simulink model "LV_grid"  (R2021b)
settings: Solver=VariableStepAuto  StartTime=0  StopTime=5.0005  FixedStep=5e-4  RelTol=1e-3
model workspace (MAT data in the model file):
  P2_1 = 3450
  idx = 1
  time_counter = 1
libraries: spsGroundLib x97, spsStairGeneratorLib x96, spsPiSectionLineLib x90, spsThreePhasePISectionLineLib x90, spsVariableInductorLib x48, spsVariableResistorLib x48, spsRMSLib x36, spsThreePhaseVIMeasurementLib x34, spsACVoltageSourceLib x5, spsLinearTransformerLib x5, spsPower3phInstantaneousLib x1, spsThreePhaseMutualInductanceZ1Z0Lib x1
(part 4 of 6)

== system LV_grid/L10/L2 ==
  Pi Section Line : spsPiSectionLineLib/Pi Section Line  LConnTagsString=__new0  RConnTagsString=__new0  Phases=1  PiSections=1  Length=0.0025  Frequency=50  Resistance=0.274  Inductance=0.073  Capacitance=12.74e-9  Measurements=None  Measurements2=None
      settings: SourceProductBaseCode=PS
  Three-Phase PI Section Line : spsThreePhasePISectionLineLib/Three-Phase PI Section Line  LConnTagsString=a|b|c  RConnTagsString=A|B|C  Length=0.0025  Frequency=50  Resistances=[ 0.274 0.959]  Inductances=[ 0.073 0.079]  Capacitances=[12.74e-9 7.751e-9]
  A : PMIOPort  Side=Left
  B : PMIOPort  Port=2  Side=Left
  C : PMIOPort  Port=3  Side=Left
  N : PMIOPort  Port=4  Side=Left
  a : PMIOPort  Port=5  Side=Right
  b : PMIOPort  Port=6  Side=Right
  c : PMIOPort  Port=7  Side=Right
  n : PMIOPort  Port=8  Side=Right
  connections:
  Pi Section Line/LConn1 -- N/RConn1
  Pi Section Line/RConn1 -- n/RConn1
  C/RConn1 -- Three-Phase PI Section Line/LConn3
  B/RConn1 -- Three-Phase PI Section Line/LConn2
  A/RConn1 -- Three-Phase PI Section Line/LConn1
  Three-Phase PI Section Line/RConn3 -- c/RConn1
  Three-Phase PI Section Line/RConn2 -- b/RConn1
  Three-Phase PI Section Line/RConn1 -- a/RConn1

== system LV_grid/L11/L1 ==
  Pi Section Line : spsPiSectionLineLib/Pi Section Line  LConnTagsString=__new0  RConnTagsString=__new0  Phases=1  PiSections=1  Length=0.0025  Frequency=50  Resistance=0.274  Inductance=0.073  Capacitance=12.74e-9  Measurements=None  Measurements2=None
      settings: SourceProductBaseCode=PS
  Three-Phase PI Section Line : spsThreePhasePISectionLineLib/Three-Phase PI Section Line  LConnTagsString=a|b|c  RConnTagsString=A|B|C  Length=0.0025  Frequency=50  Resistances=[ 0.274 0.959]  Inductances=[ 0.073 0.079]  Capacitances=[12.74e-9 7.751e-9]
  A : PMIOPort  Side=Left
  B : PMIOPort  Port=2  Side=Left
  C : PMIOPort  Port=3  Side=Left
  N : PMIOPort  Port=4  Side=Left
  a : PMIOPort  Port=5  Side=Right
  b : PMIOPort  Port=6  Side=Right
  c : PMIOPort  Port=7  Side=Right
  n : PMIOPort  Port=8  Side=Right
  connections:
  Pi Section Line/LConn1 -- N/RConn1
  Pi Section Line/RConn1 -- n/RConn1
  C/RConn1 -- Three-Phase PI Section Line/LConn3
  B/RConn1 -- Three-Phase PI Section Line/LConn2
  A/RConn1 -- Three-Phase PI Section Line/LConn1
  Three-Phase PI Section Line/RConn3 -- c/RConn1
  Three-Phase PI Section Line/RConn2 -- b/RConn1
  Three-Phase PI Section Line/RConn1 -- a/RConn1

== system LV_grid/L11/L2 ==
  Pi Section Line : spsPiSectionLineLib/Pi Section Line  LConnTagsString=__new0  RConnTagsString=__new0  Phases=1  PiSections=1  Length=0.0025  Frequency=50  Resistance=0.274  Inductance=0.073  Capacitance=12.74e-9  Measurements=None  Measurements2=None
      settings: SourceProductBaseCode=PS
  Three-Phase PI Section Line : spsThreePhasePISectionLineLib/Three-Phase PI Section Line  LConnTagsString=a|b|c  RConnTagsString=A|B|C  Length=0.0025  Frequency=50  Resistances=[ 0.274 0.959]  Inductances=[ 0.073 0.079]  Capacitances=[12.74e-9 7.751e-9]
  A : PMIOPort  Side=Left
  B : PMIOPort  Port=2  Side=Left
  C : PMIOPort  Port=3  Side=Left
  N : PMIOPort  Port=4  Side=Left
  a : PMIOPort  Port=5  Side=Right
  b : PMIOPort  Port=6  Side=Right
  c : PMIOPort  Port=7  Side=Right
  n : PMIOPort  Port=8  Side=Right
  connections:
  Pi Section Line/LConn1 -- N/RConn1
  Pi Section Line/RConn1 -- n/RConn1
  C/RConn1 -- Three-Phase PI Section Line/LConn3
  B/RConn1 -- Three-Phase PI Section Line/LConn2
  A/RConn1 -- Three-Phase PI Section Line/LConn1
  Three-Phase PI Section Line/RConn3 -- c/RConn1
  Three-Phase PI Section Line/RConn2 -- b/RConn1
  Three-Phase PI Section Line/RConn1 -- a/RConn1

== system LV_grid/L12/L1 ==
  Pi Section Line : spsPiSectionLineLib/Pi Section Line  LConnTagsString=__new0  RConnTagsString=__new0  Phases=1  PiSections=1  Length=0.0025  Frequency=50  Resistance=0.274  Inductance=0.073  Capacitance=12.74e-9  Measurements=None  Measurements2=None
      settings: SourceProductBaseCode=PS
  Three-Phase PI Section Line : spsThreePhasePISectionLineLib/Three-Phase PI Section Line  LConnTagsString=a|b|c  RConnTagsString=A|B|C  Length=0.0025  Frequency=50  Resistances=[ 0.274 0.959]  Inductances=[ 0.073 0.079]  Capacitances=[12.74e-9 7.751e-9]
  A : PMIOPort  Side=Left
  B : PMIOPort  Port=2  Side=Left
  C : PMIOPort  Port=3  Side=Left
  N : PMIOPort  Port=4  Side=Left
  a : PMIOPort  Port=5  Side=Right
  b : PMIOPort  Port=6  Side=Right
  c : PMIOPort  Port=7  Side=Right
  n : PMIOPort  Port=8  Side=Right
  connections:
  Pi Section Line/LConn1 -- N/RConn1
  Pi Section Line/RConn1 -- n/RConn1
  C/RConn1 -- Three-Phase PI Section Line/LConn3
  B/RConn1 -- Three-Phase PI Section Line/LConn2
  A/RConn1 -- Three-Phase PI Section Line/LConn1
  Three-Phase PI Section Line/RConn3 -- c/RConn1
  Three-Phase PI Section Line/RConn2 -- b/RConn1
  Three-Phase PI Section Line/RConn1 -- a/RConn1

== system LV_grid/L12/L2 ==
  Pi Section Line : spsPiSectionLineLib/Pi Section Line  LConnTagsString=__new0  RConnTagsString=__new0  Phases=1  PiSections=1  Length=0.0025  Frequency=50  Resistance=0.274  Inductance=0.073  Capacitance=12.74e-9  Measurements=None  Measurements2=None
      settings: SourceProductBaseCode=PS
  Three-Phase PI Section Line : spsThreePhasePISectionLineLib/Three-Phase PI Section Line  LConnTagsString=a|b|c  RConnTagsString=A|B|C  Length=0.0025  Frequency=50  Resistances=[ 0.274 0.959]  Inductances=[ 0.073 0.079]  Capacitances=[12.74e-9 7.751e-9]
  A : PMIOPort  Side=Left
  B : PMIOPort  Port=2  Side=Left
  C : PMIOPort  Port=3  Side=Left
  N : PMIOPort  Port=4  Side=Left
  a : PMIOPort  Port=5  Side=Right
  b : PMIOPort  Port=6  Side=Right
  c : PMIOPort  Port=7  Side=Right
  n : PMIOPort  Port=8  Side=Right
  connections:
  Pi Section Line/LConn1 -- N/RConn1
  Pi Section Line/RConn1 -- n/RConn1
  C/RConn1 -- Three-Phase PI Section Line/LConn3
  B/RConn1 -- Three-Phase PI Section Line/LConn2
  A/RConn1 -- Three-Phase PI Section Line/LConn1
  Three-Phase PI Section Line/RConn3 -- c/RConn1
  Three-Phase PI Section Line/RConn2 -- b/RConn1
  Three-Phase PI Section Line/RConn1 -- a/RConn1

== system LV_grid/L12/L3 ==
  Pi Section Line : spsPiSectionLineLib/Pi Section Line  LConnTagsString=__new0  RConnTagsString=__new0  Phases=1  PiSections=1  Length=0.0025  Frequency=50  Resistance=0.274  Inductance=0.073  Capacitance=12.74e-9  Measurements=None  Measurements2=None
      settings: SourceProductBaseCode=PS
  Three-Phase PI Section Line : spsThreePhasePISectionLineLib/Three-Phase PI Section Line  LConnTagsString=a|b|c  RConnTagsString=A|B|C  Length=0.0025  Frequency=50  Resistances=[ 0.274 0.959]  Inductances=[ 0.073 0.079]  Capacitances=[12.74e-9 7.751e-9]
  A : PMIOPort  Side=Left
  B : PMIOPort  Port=2  Side=Left
  C : PMIOPort  Port=3  Side=Left
  N : PMIOPort  Port=4  Side=Left
  a : PMIOPort  Port=5  Side=Right
  b : PMIOPort  Port=6  Side=Right
  c : PMIOPort  Port=7  Side=Right
  n : PMIOPort  Port=8  Side=Right
  connections:
  Pi Section Line/LConn1 -- N/RConn1
  Pi Section Line/RConn1 -- n/RConn1
  C/RConn1 -- Three-Phase PI Section Line/LConn3
  B/RConn1 -- Three-Phase PI Section Line/LConn2
  A/RConn1 -- Three-Phase PI Section Line/LConn1
  Three-Phase PI Section Line/RConn3 -- c/RConn1
  Three-Phase PI Section Line/RConn2 -- b/RConn1
  Three-Phase PI Section Line/RConn1 -- a/RConn1

== system LV_grid/L12/L4 ==
  Pi Section Line : spsPiSectionLineLib/Pi Section Line  LConnTagsString=__new0  RConnTagsString=__new0  Phases=1  PiSections=1  Length=0.0025  Frequency=50  Resistance=0.274  Inductance=0.073  Capacitance=12.74e-9  Measurements=None  Measurements2=None
      settings: SourceProductBaseCode=PS
  Three-Phase PI Section Line : spsThreePhasePISectionLineLib/Three-Phase PI Section Line  LConnTagsString=a|b|c  RConnTagsString=A|B|C  Length=0.0025  Frequency=50  Resistances=[ 0.274 0.959]  Inductances=[ 0.073 0.079]  Capacitances=[12.74e-9 7.751e-9]
  A : PMIOPort  Side=Left
  B : PMIOPort  Port=2  Side=Left
  C : PMIOPort  Port=3  Side=Left
  N : PMIOPort  Port=4  Side=Left
  a : PMIOPort  Port=5  Side=Right
  b : PMIOPort  Port=6  Side=Right
  c : PMIOPort  Port=7  Side=Right
  n : PMIOPort  Port=8  Side=Right
  connections:
  Pi Section Line/LConn1 -- N/RConn1
  Pi Section Line/RConn1 -- n/RConn1
  C/RConn1 -- Three-Phase PI Section Line/LConn3
  B/RConn1 -- Three-Phase PI Section Line/LConn2
  A/RConn1 -- Three-Phase PI Section Line/LConn1
  Three-Phase PI Section Line/RConn3 -- c/RConn1
  Three-Phase PI Section Line/RConn2 -- b/RConn1
  Three-Phase PI Section Line/RConn1 -- a/RConn1

== system LV_grid/L12/L5 ==
  Pi Section Line : spsPiSectionLineLib/Pi Section Line  LConnTagsString=__new0  RConnTagsString=__new0  Phases=1  PiSections=1  Length=0.0025  Frequency=50  Resistance=0.274  Inductance=0.073  Capacitance=12.74e-9  Measurements=None  Measurements2=None
      settings: SourceProductBaseCode=PS
  Three-Phase PI Section Line : spsThreePhasePISectionLineLib/Three-Phase PI Section Line  LConnTagsString=a|b|c  RConnTagsString=A|B|C  Length=0.0025  Frequency=50  Resistances=[ 0.274 0.959]  Inductances=[ 0.073 0.079]  Capacitances=[12.74e-9 7.751e-9]
  A : PMIOPort  Side=Left
  B : PMIOPort  Port=2  Side=Left
  C : PMIOPort  Port=3  Side=Left
  N : PMIOPort  Port=4  Side=Left
  a : PMIOPort  Port=5  Side=Right
  b : PMIOPort  Port=6  Side=Right
  c : PMIOPort  Port=7  Side=Right
  n : PMIOPort  Port=8  Side=Right
  connections:
  Pi Section Line/LConn1 -- N/RConn1
  Pi Section Line/RConn1 -- n/RConn1
  C/RConn1 -- Three-Phase PI Section Line/LConn3
  B/RConn1 -- Three-Phase PI Section Line/LConn2
  A/RConn1 -- Three-Phase PI Section Line/LConn1
  Three-Phase PI Section Line/RConn3 -- c/RConn1
  Three-Phase PI Section Line/RConn2 -- b/RConn1
  Three-Phase PI Section Line/RConn1 -- a/RConn1

== system LV_grid/L13/L1 ==
  Pi Section Line : spsPiSectionLineLib/Pi Section Line  LConnTagsString=__new0  RConnTagsString=__new0  Phases=1  PiSections=1  Length=0.0025  Frequency=50  Resistance=0.274  Inductance=0.073  Capacitance=12.74e-9  Measurements=None  Measurements2=None
      settings: SourceProductBaseCode=PS
  Three-Phase PI Section Line : spsThreePhasePISectionLineLib/Three-Phase PI Section Line  LConnTagsString=a|b|c  RConnTagsString=A|B|C  Length=0.0025  Frequency=50  Resistances=[ 0.274 0.959]  Inductances=[ 0.073 0.079]  Capacitances=[12.74e-9 7.751e-9]
  A : PMIOPort  Side=Left
  B : PMIOPort  Port=2  Side=Left
  C : PMIOPort  Port=3  Side=Left
  N : PMIOPort  Port=4  Side=Left
  a : PMIOPort  Port=5  Side=Right
  b : PMIOPort  Port=6  Side=Right
  c : PMIOPort  Port=7  Side=Right
  n : PMIOPort  Port=8  Side=Right
  connections:
  Pi Section Line/LConn1 -- N/RConn1
  Pi Section Line/RConn1 -- n/RConn1
  C/RConn1 -- Three-Phase PI Section Line/LConn3
  B/RConn1 -- Three-Phase PI Section Line/LConn2
  A/RConn1 -- Three-Phase PI Section Line/LConn1
  Three-Phase PI Section Line/RConn3 -- c/RConn1
  Three-Phase PI Section Line/RConn2 -- b/RConn1
  Three-Phase PI Section Line/RConn1 -- a/RConn1

== system LV_grid/L13/L2 ==
  Pi Section Line : spsPiSectionLineLib/Pi Section Line  LConnTagsString=__new0  RConnTagsString=__new0  Phases=1  PiSections=1  Length=0.0025  Frequency=50  Resistance=0.274  Inductance=0.073  Capacitance=12.74e-9  Measurements=None  Measurements2=None
      settings: SourceProductBaseCode=PS
  Three-Phase PI Section Line : spsThreePhasePISectionLineLib/Three-Phase PI Section Line  LConnTagsString=a|b|c  RConnTagsString=A|B|C  Length=0.0025  Frequency=50  Resistances=[ 0.274 0.959]  Inductances=[ 0.073 0.079]  Capacitances=[12.74e-9 7.751e-9]
  A : PMIOPort  Side=Left
  B : PMIOPort  Port=2  Side=Left
  C : PMIOPort  Port=3  Side=Left
  N : PMIOPort  Port=4  Side=Left
  a : PMIOPort  Port=5  Side=Right
  b : PMIOPort  Port=6  Side=Right
  c : PMIOPort  Port=7  Side=Right
  n : PMIOPort  Port=8  Side=Right
  connections:
  Pi Section Line/LConn1 -- N/RConn1
  Pi Section Line/RConn1 -- n/RConn1
  C/RConn1 -- Three-Phase PI Section Line/LConn3
  B/RConn1 -- Three-Phase PI Section Line/LConn2
  A/RConn1 -- Three-Phase PI Section Line/LConn1
  Three-Phase PI Section Line/RConn3 -- c/RConn1
  Three-Phase PI Section Line/RConn2 -- b/RConn1
  Three-Phase PI Section Line/RConn1 -- a/RConn1

== system LV_grid/L14/L1 ==
  Pi Section Line : spsPiSectionLineLib/Pi Section Line  LConnTagsString=__new0  RConnTagsString=__new0  Phases=1  PiSections=1  Length=0.0025  Frequency=50  Resistance=0.274  Inductance=0.073  Capacitance=12.74e-9  Measurements=None  Measurements2=None
      settings: SourceProductBaseCode=PS
  Three-Phase PI Section Line : spsThreePhasePISectionLineLib/Three-Phase PI Section Line  LConnTagsString=a|b|c  RConnTagsString=A|B|C  Length=0.0025  Frequency=50  Resistances=[ 0.274 0.959]  Inductances=[ 0.073 0.079]  Capacitances=[12.74e-9 7.751e-9]
  A : PMIOPort  Side=Left
  B : PMIOPort  Port=2  Side=Left
  C : PMIOPort  Port=3  Side=Left
  N : PMIOPort  Port=4  Side=Left
  a : PMIOPort  Port=5  Side=Right
  b : PMIOPort  Port=6  Side=Right
  c : PMIOPort  Port=7  Side=Right
  n : PMIOPort  Port=8  Side=Right
  connections:
  Pi Section Line/LConn1 -- N/RConn1
  Pi Section Line/RConn1 -- n/RConn1
  C/RConn1 -- Three-Phase PI Section Line/LConn3
  B/RConn1 -- Three-Phase PI Section Line/LConn2
  A/RConn1 -- Three-Phase PI Section Line/LConn1
  Three-Phase PI Section Line/RConn3 -- c/RConn1
  Three-Phase PI Section Line/RConn2 -- b/RConn1
  Three-Phase PI Section Line/RConn1 -- a/RConn1

== system LV_grid/L15/L1 ==
  Pi Section Line : spsPiSectionLineLib/Pi Section Line  LConnTagsString=__new0  RConnTagsString=__new0  Phases=1  PiSections=1  Length=0.0025  Frequency=50  Resistance=0.274  Inductance=0.073  Capacitance=12.74e-9  Measurements=None  Measurements2=None
      settings: SourceProductBaseCode=PS
  Three-Phase PI Section Line : spsThreePhasePISectionLineLib/Three-Phase PI Section Line  LConnTagsString=a|b|c  RConnTagsString=A|B|C  Length=0.0025  Frequency=50  Resistances=[ 0.274 0.959]  Inductances=[ 0.073 0.079]  Capacitances=[12.74e-9 7.751e-9]
  A : PMIOPort  Side=Left
  B : PMIOPort  Port=2  Side=Left
  C : PMIOPort  Port=3  Side=Left
  N : PMIOPort  Port=4  Side=Left
  a : PMIOPort  Port=5  Side=Right
  b : PMIOPort  Port=6  Side=Right
  c : PMIOPort  Port=7  Side=Right
  n : PMIOPort  Port=8  Side=Right
  connections:
  Pi Section Line/LConn1 -- N/RConn1
  Pi Section Line/RConn1 -- n/RConn1
  C/RConn1 -- Three-Phase PI Section Line/LConn3
  B/RConn1 -- Three-Phase PI Section Line/LConn2
  A/RConn1 -- Three-Phase PI Section Line/LConn1
  Three-Phase PI Section Line/RConn3 -- c/RConn1
  Three-Phase PI Section Line/RConn2 -- b/RConn1
  Three-Phase PI Section Line/RConn1 -- a/RConn1

== system LV_grid/L15/L2 ==
  Pi Section Line : spsPiSectionLineLib/Pi Section Line  LConnTagsString=__new0  RConnTagsString=__new0  Phases=1  PiSections=1  Length=0.0025  Frequency=50  Resistance=0.274  Inductance=0.073  Capacitance=12.74e-9  Measurements=None  Measurements2=None
      settings: SourceProductBaseCode=PS
  Three-Phase PI Section Line : spsThreePhasePISectionLineLib/Three-Phase PI Section Line  LConnTagsString=a|b|c  RConnTagsString=A|B|C  Length=0.0025  Frequency=50  Resistances=[ 0.274 0.959]  Inductances=[ 0.073 0.079]  Capacitances=[12.74e-9 7.751e-9]
  A : PMIOPort  Side=Left
  B : PMIOPort  Port=2  Side=Left
  C : PMIOPort  Port=3  Side=Left
  N : PMIOPort  Port=4  Side=Left
  a : PMIOPort  Port=5  Side=Right
  b : PMIOPort  Port=6  Side=Right
  c : PMIOPort  Port=7  Side=Right
  n : PMIOPort  Port=8  Side=Right
  connections:
  Pi Section Line/LConn1 -- N/RConn1
  Pi Section Line/RConn1 -- n/RConn1
  C/RConn1 -- Three-Phase PI Section Line/LConn3
  B/RConn1 -- Three-Phase PI Section Line/LConn2
  A/RConn1 -- Three-Phase PI Section Line/LConn1
  Three-Phase PI Section Line/RConn3 -- c/RConn1
  Three-Phase PI Section Line/RConn2 -- b/RConn1
  Three-Phase PI Section Line/RConn1 -- a/RConn1

== system LV_grid/L16/L1 ==
  Pi Section Line : spsPiSectionLineLib/Pi Section Line  LConnTagsString=__new0  RConnTagsString=__new0  Phases=1  PiSections=1  Length=0.0025  Frequency=50  Resistance=0.274  Inductance=0.073  Capacitance=12.74e-9  Measurements=None  Measurements2=None
      settings: SourceProductBaseCode=PS
  Three-Phase PI Section Line : spsThreePhasePISectionLineLib/Three-Phase PI Section Line  LConnTagsString=a|b|c  RConnTagsString=A|B|C  Length=0.0025  Frequency=50  Resistances=[ 0.274 0.959]  Inductances=[ 0.073 0.079]  Capacitances=[12.74e-9 7.751e-9]
  A : PMIOPort  Side=Left
  B : PMIOPort  Port=2  Side=Left
  C : PMIOPort  Port=3  Side=Left
  N : PMIOPort  Port=4  Side=Left
  a : PMIOPort  Port=5  Side=Right
  b : PMIOPort  Port=6  Side=Right
  c : PMIOPort  Port=7  Side=Right
  n : PMIOPort  Port=8  Side=Right
  connections:
  Pi Section Line/LConn1 -- N/RConn1
  Pi Section Line/RConn1 -- n/RConn1
  C/RConn1 -- Three-Phase PI Section Line/LConn3
  B/RConn1 -- Three-Phase PI Section Line/LConn2
  A/RConn1 -- Three-Phase PI Section Line/LConn1
  Three-Phase PI Section Line/RConn3 -- c/RConn1
  Three-Phase PI Section Line/RConn2 -- b/RConn1
  Three-Phase PI Section Line/RConn1 -- a/RConn1

== system LV_grid/L17/L1 ==
  Pi Section Line : spsPiSectionLineLib/Pi Section Line  LConnTagsString=__new0  RConnTagsString=__new0  Phases=1  PiSections=1  Length=0.0025  Frequency=50  Resistance=0.274  Inductance=0.073  Capacitance=12.74e-9  Measurements=None  Measurements2=None
      settings: SourceProductBaseCode=PS
  Three-Phase PI Section Line : spsThreePhasePISectionLineLib/Three-Phase PI Section Line  LConnTagsString=a|b|c  RConnTagsString=A|B|C  Length=0.0025  Frequency=50  Resistances=[ 0.274 0.959]  Inductances=[ 0.073 0.079]  Capacitances=[12.74e-9 7.751e-9]
  A : PMIOPort  Side=Left
  B : PMIOPort  Port=2  Side=Left
  C : PMIOPort  Port=3  Side=Left
  N : PMIOPort  Port=4  Side=Left
  a : PMIOPort  Port=5  Side=Right
  b : PMIOPort  Port=6  Side=Right
  c : PMIOPort  Port=7  Side=Right
  n : PMIOPort  Port=8  Side=Right
  connections:
  Pi Section Line/LConn1 -- N/RConn1
  Pi Section Line/RConn1 -- n/RConn1
  C/RConn1 -- Three-Phase PI Section Line/LConn3
  B/RConn1 -- Three-Phase PI Section Line/LConn2
  A/RConn1 -- Three-Phase PI Section Line/LConn1
  Three-Phase PI Section Line/RConn3 -- c/RConn1
  Three-Phase PI Section Line/RConn2 -- b/RConn1
  Three-Phase PI Section Line/RConn1 -- a/RConn1

== system LV_grid/L17/L2 ==
  Pi Section Line : spsPiSectionLineLib/Pi Section Line  LConnTagsString=__new0  RConnTagsString=__new0  Phases=1  PiSections=1  Length=0.0025  Frequency=50  Resistance=0.274  Inductance=0.073  Capacitance=12.74e-9  Measurements=None  Measurements2=None
      settings: SourceProductBaseCode=PS
  Three-Phase PI Section Line : spsThreePhasePISectionLineLib/Three-Phase PI Section Line  LConnTagsString=a|b|c  RConnTagsString=A|B|C  Length=0.0025  Frequency=50  Resistances=[ 0.274 0.959]  Inductances=[ 0.073 0.079]  Capacitances=[12.74e-9 7.751e-9]
  A : PMIOPort  Side=Left
  B : PMIOPort  Port=2  Side=Left
  C : PMIOPort  Port=3  Side=Left
  N : PMIOPort  Port=4  Side=Left
  a : PMIOPort  Port=5  Side=Right
  b : PMIOPort  Port=6  Side=Right
  c : PMIOPort  Port=7  Side=Right
  n : PMIOPort  Port=8  Side=Right
  connections:
  Pi Section Line/LConn1 -- N/RConn1
  Pi Section Line/RConn1 -- n/RConn1
  C/RConn1 -- Three-Phase PI Section Line/LConn3
  B/RConn1 -- Three-Phase PI Section Line/LConn2
  A/RConn1 -- Three-Phase PI Section Line/LConn1
  Three-Phase PI Section Line/RConn3 -- c/RConn1
  Three-Phase PI Section Line/RConn2 -- b/RConn1
  Three-Phase PI Section Line/RConn1 -- a/RConn1

== system LV_grid/L17/L3 ==
  Pi Section Line : spsPiSectionLineLib/Pi Section Line  LConnTagsString=__new0  RConnTagsString=__new0  Phases=1  PiSections=1  Length=0.0025  Frequency=50  Resistance=0.274  Inductance=0.073  Capacitance=12.74e-9  Measurements=None  Measurements2=None
      settings: SourceProductBaseCode=PS
  Three-Phase PI Section Line : spsThreePhasePISectionLineLib/Three-Phase PI Section Line  LConnTagsString=a|b|c  RConnTagsString=A|B|C  Length=0.0025  Frequency=50  Resistances=[ 0.274 0.959]  Inductances=[ 0.073 0.079]  Capacitances=[12.74e-9 7.751e-9]
  A : PMIOPort  Side=Left
  B : PMIOPort  Port=2  Side=Left
  C : PMIOPort  Port=3  Side=Left
  N : PMIOPort  Port=4  Side=Left
  a : PMIOPort  Port=5  Side=Right
  b : PMIOPort  Port=6  Side=Right
  c : PMIOPort  Port=7  Side=Right
  n : PMIOPort  Port=8  Side=Right
  connections:
  Pi Section Line/LConn1 -- N/RConn1
  Pi Section Line/RConn1 -- n/RConn1
  C/RConn1 -- Three-Phase PI Section Line/LConn3
  B/RConn1 -- Three-Phase PI Section Line/LConn2
  A/RConn1 -- Three-Phase PI Section Line/LConn1
  Three-Phase PI Section Line/RConn3 -- c/RConn1
  Three-Phase PI Section Line/RConn2 -- b/RConn1
  Three-Phase PI Section Line/RConn1 -- a/RConn1

== system LV_grid/L18/L1 ==
  Pi Section Line : spsPiSectionLineLib/Pi Section Line  LConnTagsString=__new0  RConnTagsString=__new0  Phases=1  PiSections=1  Length=0.0025  Frequency=50  Resistance=0.274  Inductance=0.073  Capacitance=12.74e-9  Measurements=None  Measurements2=None
      settings: SourceProductBaseCode=PS
  Three-Phase PI Section Line : spsThreePhasePISectionLineLib/Three-Phase PI Section Line  LConnTagsString=a|b|c  RConnTagsString=A|B|C  Length=0.0025  Frequency=50  Resistances=[ 0.274 0.959]  Inductances=[ 0.073 0.079]  Capacitances=[12.74e-9 7.751e-9]
  A : PMIOPort  Side=Left
  B : PMIOPort  Port=2  Side=Left
  C : PMIOPort  Port=3  Side=Left
  N : PMIOPort  Port=4  Side=Left
  a : PMIOPort  Port=5  Side=Right
  b : PMIOPort  Port=6  Side=Right
  c : PMIOPort  Port=7  Side=Right
  n : PMIOPort  Port=8  Side=Right
  connections:
  Pi Section Line/LConn1 -- N/RConn1
  Pi Section Line/RConn1 -- n/RConn1
  C/RConn1 -- Three-Phase PI Section Line/LConn3
  B/RConn1 -- Three-Phase PI Section Line/LConn2
  A/RConn1 -- Three-Phase PI Section Line/LConn1
  Three-Phase PI Section Line/RConn3 -- c/RConn1
  Three-Phase PI Section Line/RConn2 -- b/RConn1
  Three-Phase PI Section Line/RConn1 -- a/RConn1

== system LV_grid/L18/L2 ==
  Pi Section Line : spsPiSectionLineLib/Pi Section Line  LConnTagsString=__new0  RConnTagsString=__new0  Phases=1  PiSections=1  Length=0.0025  Frequency=50  Resistance=0.274  Inductance=0.073  Capacitance=12.74e-9  Measurements=None  Measurements2=None
      settings: SourceProductBaseCode=PS
  Three-Phase PI Section Line : spsThreePhasePISectionLineLib/Three-Phase PI Section Line  LConnTagsString=a|b|c  RConnTagsString=A|B|C  Length=0.0025  Frequency=50  Resistances=[ 0.274 0.959]  Inductances=[ 0.073 0.079]  Capacitances=[12.74e-9 7.751e-9]
  A : PMIOPort  Side=Left
  B : PMIOPort  Port=2  Side=Left
  C : PMIOPort  Port=3  Side=Left
  N : PMIOPort  Port=4  Side=Left
  a : PMIOPort  Port=5  Side=Right
  b : PMIOPort  Port=6  Side=Right
  c : PMIOPort  Port=7  Side=Right
  n : PMIOPort  Port=8  Side=Right
  connections:
  Pi Section Line/LConn1 -- N/RConn1
  Pi Section Line/RConn1 -- n/RConn1
  C/RConn1 -- Three-Phase PI Section Line/LConn3
  B/RConn1 -- Three-Phase PI Section Line/LConn2
  A/RConn1 -- Three-Phase PI Section Line/LConn1
  Three-Phase PI Section Line/RConn3 -- c/RConn1
  Three-Phase PI Section Line/RConn2 -- b/RConn1
  Three-Phase PI Section Line/RConn1 -- a/RConn1

== system LV_grid/L19/L1 ==
  Pi Section Line : spsPiSectionLineLib/Pi Section Line  LConnTagsString=__new0  RConnTagsString=__new0  Phases=1  PiSections=1  Length=0.0025  Frequency=50  Resistance=0.274  Inductance=0.073  Capacitance=12.74e-9  Measurements=None  Measurements2=None
      settings: SourceProductBaseCode=PS
  Three-Phase PI Section Line : spsThreePhasePISectionLineLib/Three-Phase PI Section Line  LConnTagsString=a|b|c  RConnTagsString=A|B|C  Length=0.0025  Frequency=50  Resistances=[ 0.274 0.959]  Inductances=[ 0.073 0.079]  Capacitances=[12.74e-9 7.751e-9]
  A : PMIOPort  Side=Left
  B : PMIOPort  Port=2  Side=Left
  C : PMIOPort  Port=3  Side=Left
  N : PMIOPort  Port=4  Side=Left
  a : PMIOPort  Port=5  Side=Right
  b : PMIOPort  Port=6  Side=Right
  c : PMIOPort  Port=7  Side=Right
  n : PMIOPort  Port=8  Side=Right
  connections:
  Pi Section Line/LConn1 -- N/RConn1
  Pi Section Line/RConn1 -- n/RConn1
  C/RConn1 -- Three-Phase PI Section Line/LConn3
  B/RConn1 -- Three-Phase PI Section Line/LConn2
  A/RConn1 -- Three-Phase PI Section Line/LConn1
  Three-Phase PI Section Line/RConn3 -- c/RConn1
  Three-Phase PI Section Line/RConn2 -- b/RConn1
  Three-Phase PI Section Line/RConn1 -- a/RConn1

== system LV_grid/L2/L1 ==
  Pi Section Line : spsPiSectionLineLib/Pi Section Line  LConnTagsString=__new0  RConnTagsString=__new0  Phases=1  PiSections=1  Length=0.0025  Frequency=50  Resistance=0.274  Inductance=0.073  Capacitance=12.74e-9  Measurements=None  Measurements2=None
      settings: SourceProductBaseCode=PS
  Three-Phase PI Section Line : spsThreePhasePISectionLineLib/Three-Phase PI Section Line  LConnTagsString=a|b|c  RConnTagsString=A|B|C  Length=0.0025  Frequency=50  Resistances=[ 0.274 0.959]  Inductances=[ 0.073 0.079]  Capacitances=[12.74e-9 7.751e-9]
  A : PMIOPort  Side=Left
  B : PMIOPort  Port=2  Side=Left
  C : PMIOPort  Port=3  Side=Left
  N : PMIOPort  Port=4  Side=Left
  a : PMIOPort  Port=5  Side=Right
  b : PMIOPort  Port=6  Side=Right
  c : PMIOPort  Port=7  Side=Right
  n : PMIOPort  Port=8  Side=Right
  connections:
  Pi Section Line/LConn1 -- N/RConn1
  Pi Section Line/RConn1 -- n/RConn1
  C/RConn1 -- Three-Phase PI Section Line/LConn3
  B/RConn1 -- Three-Phase PI Section Line/LConn2
  A/RConn1 -- Three-Phase PI Section Line/LConn1
  Three-Phase PI Section Line/RConn3 -- c/RConn1
  Three-Phase PI Section Line/RConn2 -- b/RConn1
  Three-Phase PI Section Line/RConn1 -- a/RConn1

== system LV_grid/L20/L1 ==
  Pi Section Line : spsPiSectionLineLib/Pi Section Line  LConnTagsString=__new0  RConnTagsString=__new0  Phases=1  PiSections=1  Length=0.0025  Frequency=50  Resistance=0.274  Inductance=0.073  Capacitance=12.74e-9  Measurements=None  Measurements2=None
      settings: SourceProductBaseCode=PS
  Three-Phase PI Section Line : spsThreePhasePISectionLineLib/Three-Phase PI Section Line  LConnTagsString=a|b|c  RConnTagsString=A|B|C  Length=0.0025  Frequency=50  Resistances=[ 0.274 0.959]  Inductances=[ 0.073 0.079]  Capacitances=[12.74e-9 7.751e-9]
  A : PMIOPort  Side=Left
  B : PMIOPort  Port=2  Side=Left
  C : PMIOPort  Port=3  Side=Left
  N : PMIOPort  Port=4  Side=Left
  a : PMIOPort  Port=5  Side=Right
  b : PMIOPort  Port=6  Side=Right
  c : PMIOPort  Port=7  Side=Right
  n : PMIOPort  Port=8  Side=Right
  connections:
  Pi Section Line/LConn1 -- N/RConn1
  Pi Section Line/RConn1 -- n/RConn1
  C/RConn1 -- Three-Phase PI Section Line/LConn3
  B/RConn1 -- Three-Phase PI Section Line/LConn2
  A/RConn1 -- Three-Phase PI Section Line/LConn1
  Three-Phase PI Section Line/RConn3 -- c/RConn1
  Three-Phase PI Section Line/RConn2 -- b/RConn1
  Three-Phase PI Section Line/RConn1 -- a/RConn1

== system LV_grid/L20/L2 ==
  Pi Section Line : spsPiSectionLineLib/Pi Section Line  LConnTagsString=__new0  RConnTagsString=__new0  Phases=1  PiSections=1  Length=0.0025  Frequency=50  Resistance=0.274  Inductance=0.073  Capacitance=12.74e-9  Measurements=None  Measurements2=None
      settings: SourceProductBaseCode=PS
  Three-Phase PI Section Line : spsThreePhasePISectionLineLib/Three-Phase PI Section Line  LConnTagsString=a|b|c  RConnTagsString=A|B|C  Length=0.0025  Frequency=50  Resistances=[ 0.274 0.959]  Inductances=[ 0.073 0.079]  Capacitances=[12.74e-9 7.751e-9]
  A : PMIOPort  Side=Left
  B : PMIOPort  Port=2  Side=Left
  C : PMIOPort  Port=3  Side=Left
  N : PMIOPort  Port=4  Side=Left
  a : PMIOPort  Port=5  Side=Right
  b : PMIOPort  Port=6  Side=Right
  c : PMIOPort  Port=7  Side=Right
  n : PMIOPort  Port=8  Side=Right
  connections:
  Pi Section Line/LConn1 -- N/RConn1
  Pi Section Line/RConn1 -- n/RConn1
  C/RConn1 -- Three-Phase PI Section Line/LConn3
  B/RConn1 -- Three-Phase PI Section Line/LConn2
  A/RConn1 -- Three-Phase PI Section Line/LConn1
  Three-Phase PI Section Line/RConn3 -- c/RConn1
  Three-Phase PI Section Line/RConn2 -- b/RConn1
  Three-Phase PI Section Line/RConn1 -- a/RConn1

== system LV_grid/L20/L3 ==
  Pi Section Line : spsPiSectionLineLib/Pi Section Line  LConnTagsString=__new0  RConnTagsString=__new0  Phases=1  PiSections=1  Length=0.0025  Frequency=50  Resistance=0.274  Inductance=0.073  Capacitance=12.74e-9  Measurements=None  Measurements2=None
      settings: SourceProductBaseCode=PS
  Three-Phase PI Section Line : spsThreePhasePISectionLineLib/Three-Phase PI Section Line  LConnTagsString=a|b|c  RConnTagsString=A|B|C  Length=0.0025  Frequency=50  Resistances=[ 0.274 0.959]  Inductances=[ 0.073 0.079]  Capacitances=[12.74e-9 7.751e-9]
  A : PMIOPort  Side=Left
  B : PMIOPort  Port=2  Side=Left
  C : PMIOPort  Port=3  Side=Left
  N : PMIOPort  Port=4  Side=Left
  a : PMIOPort  Port=5  Side=Right
  b : PMIOPort  Port=6  Side=Right
  c : PMIOPort  Port=7  Side=Right
  n : PMIOPort  Port=8  Side=Right
  connections:
  Pi Section Line/LConn1 -- N/RConn1
  Pi Section Line/RConn1 -- n/RConn1
  C/RConn1 -- Three-Phase PI Section Line/LConn3
  B/RConn1 -- Three-Phase PI Section Line/LConn2
  A/RConn1 -- Three-Phase PI Section Line/LConn1
  Three-Phase PI Section Line/RConn3 -- c/RConn1
  Three-Phase PI Section Line/RConn2 -- b/RConn1
  Three-Phase PI Section Line/RConn1 -- a/RConn1

== system LV_grid/L21/L1 ==
  Pi Section Line : spsPiSectionLineLib/Pi Section Line  LConnTagsString=__new0  RConnTagsString=__new0  Phases=1  PiSections=1  Length=0.0025  Frequency=50  Resistance=0.274  Inductance=0.073  Capacitance=12.74e-9  Measurements=None  Measurements2=None
      settings: SourceProductBaseCode=PS
  Three-Phase PI Section Line : spsThreePhasePISectionLineLib/Three-Phase PI Section Line  LConnTagsString=a|b|c  RConnTagsString=A|B|C  Length=0.0025  Frequency=50  Resistances=[ 0.274 0.959]  Inductances=[ 0.073 0.079]  Capacitances=[12.74e-9 7.751e-9]
  A : PMIOPort  Side=Left
  B : PMIOPort  Port=2  Side=Left
  C : PMIOPort  Port=3  Side=Left
  N : PMIOPort  Port=4  Side=Left
  a : PMIOPort  Port=5  Side=Right
  b : PMIOPort  Port=6  Side=Right
  c : PMIOPort  Port=7  Side=Right
  n : PMIOPort  Port=8  Side=Right
  connections:
  Pi Section Line/LConn1 -- N/RConn1
  Pi Section Line/RConn1 -- n/RConn1
  C/RConn1 -- Three-Phase PI Section Line/LConn3
  B/RConn1 -- Three-Phase PI Section Line/LConn2
  A/RConn1 -- Three-Phase PI Section Line/LConn1
  Three-Phase PI Section Line/RConn3 -- c/RConn1
  Three-Phase PI Section Line/RConn2 -- b/RConn1
  Three-Phase PI Section Line/RConn1 -- a/RConn1

== system LV_grid/L21/L2 ==
  Pi Section Line : spsPiSectionLineLib/Pi Section Line  LConnTagsString=__new0  RConnTagsString=__new0  Phases=1  PiSections=1  Length=0.0025  Frequency=50  Resistance=0.274  Inductance=0.073  Capacitance=12.74e-9  Measurements=None  Measurements2=None
      settings: SourceProductBaseCode=PS
  Three-Phase PI Section Line : spsThreePhasePISectionLineLib/Three-Phase PI Section Line  LConnTagsString=a|b|c  RConnTagsString=A|B|C  Length=0.0025  Frequency=50  Resistances=[ 0.274 0.959]  Inductances=[ 0.073 0.079]  Capacitances=[12.74e-9 7.751e-9]
  A : PMIOPort  Side=Left
  B : PMIOPort  Port=2  Side=Left
  C : PMIOPort  Port=3  Side=Left
  N : PMIOPort  Port=4  Side=Left
  a : PMIOPort  Port=5  Side=Right
  b : PMIOPort  Port=6  Side=Right
  c : PMIOPort  Port=7  Side=Right
  n : PMIOPort  Port=8  Side=Right
  connections:
  Pi Section Line/LConn1 -- N/RConn1
  Pi Section Line/RConn1 -- n/RConn1
  C/RConn1 -- Three-Phase PI Section Line/LConn3
  B/RConn1 -- Three-Phase PI Section Line/LConn2
  A/RConn1 -- Three-Phase PI Section Line/LConn1
  Three-Phase PI Section Line/RConn3 -- c/RConn1
  Three-Phase PI Section Line/RConn2 -- b/RConn1
  Three-Phase PI Section Line/RConn1 -- a/RConn1

== system LV_grid/L21/L3 ==
  Pi Section Line : spsPiSectionLineLib/Pi Section Line  LConnTagsString=__new0  RConnTagsString=__new0  Phases=1  PiSections=1  Length=0.0025  Frequency=50  Resistance=0.274  Inductance=0.073  Capacitance=12.74e-9  Measurements=None  Measurements2=None
      settings: SourceProductBaseCode=PS
  Three-Phase PI Section Line : spsThreePhasePISectionLineLib/Three-Phase PI Section Line  LConnTagsString=a|b|c  RConnTagsString=A|B|C  Length=0.0025  Frequency=50  Resistances=[ 0.274 0.959]  Inductances=[ 0.073 0.079]  Capacitances=[12.74e-9 7.751e-9]
  A : PMIOPort  Side=Left
  B : PMIOPort  Port=2  Side=Left
  C : PMIOPort  Port=3  Side=Left
  N : PMIOPort  Port=4  Side=Left
  a : PMIOPort  Port=5  Side=Right
  b : PMIOPort  Port=6  Side=Right
  c : PMIOPort  Port=7  Side=Right
  n : PMIOPort  Port=8  Side=Right
  connections:
  Pi Section Line/LConn1 -- N/RConn1
  Pi Section Line/RConn1 -- n/RConn1
  C/RConn1 -- Three-Phase PI Section Line/LConn3
  B/RConn1 -- Three-Phase PI Section Line/LConn2
  A/RConn1 -- Three-Phase PI Section Line/LConn1
  Three-Phase PI Section Line/RConn3 -- c/RConn1
  Three-Phase PI Section Line/RConn2 -- b/RConn1
  Three-Phase PI Section Line/RConn1 -- a/RConn1

== system LV_grid/L21/L4 ==
  Pi Section Line : spsPiSectionLineLib/Pi Section Line  LConnTagsString=__new0  RConnTagsString=__new0  Phases=1  PiSections=1  Length=0.0025  Frequency=50  Resistance=0.274  Inductance=0.073  Capacitance=12.74e-9  Measurements=None  Measurements2=None
      settings: SourceProductBaseCode=PS
  Three-Phase PI Section Line : spsThreePhasePISectionLineLib/Three-Phase PI Section Line  LConnTagsString=a|b|c  RConnTagsString=A|B|C  Length=0.0025  Frequency=50  Resistances=[ 0.274 0.959]  Inductances=[ 0.073 0.079]  Capacitances=[12.74e-9 7.751e-9]
  A : PMIOPort  Side=Left
  B : PMIOPort  Port=2  Side=Left
  C : PMIOPort  Port=3  Side=Left
  N : PMIOPort  Port=4  Side=Left
  a : PMIOPort  Port=5  Side=Right
  b : PMIOPort  Port=6  Side=Right
  c : PMIOPort  Port=7  Side=Right
  n : PMIOPort  Port=8  Side=Right
  connections:
  Pi Section Line/LConn1 -- N/RConn1
  Pi Section Line/RConn1 -- n/RConn1
  C/RConn1 -- Three-Phase PI Section Line/LConn3
  B/RConn1 -- Three-Phase PI Section Line/LConn2
  A/RConn1 -- Three-Phase PI Section Line/LConn1
  Three-Phase PI Section Line/RConn3 -- c/RConn1
  Three-Phase PI Section Line/RConn2 -- b/RConn1
  Three-Phase PI Section Line/RConn1 -- a/RConn1

== system LV_grid/L21/L5 ==
  Pi Section Line : spsPiSectionLineLib/Pi Section Line  LConnTagsString=__new0  RConnTagsString=__new0  Phases=1  PiSections=1  Length=0.0025  Frequency=50  Resistance=0.274  Inductance=0.073  Capacitance=12.74e-9  Measurements=None  Measurements2=None
      settings: SourceProductBaseCode=PS
  Three-Phase PI Section Line : spsThreePhasePISectionLineLib/Three-Phase PI Section Line  LConnTagsString=a|b|c  RConnTagsString=A|B|C  Length=0.0025  Frequency=50  Resistances=[ 0.274 0.959]  Inductances=[ 0.073 0.079]  Capacitances=[12.74e-9 7.751e-9]
  A : PMIOPort  Side=Left
  B : PMIOPort  Port=2  Side=Left
  C : PMIOPort  Port=3  Side=Left
  N : PMIOPort  Port=4  Side=Left
  a : PMIOPort  Port=5  Side=Right
  b : PMIOPort  Port=6  Side=Right
  c : PMIOPort  Port=7  Side=Right
  n : PMIOPort  Port=8  Side=Right
  connections:
  Pi Section Line/LConn1 -- N/RConn1
  Pi Section Line/RConn1 -- n/RConn1
  C/RConn1 -- Three-Phase PI Section Line/LConn3
  B/RConn1 -- Three-Phase PI Section Line/LConn2
  A/RConn1 -- Three-Phase PI Section Line/LConn1
  Three-Phase PI Section Line/RConn3 -- c/RConn1
  Three-Phase PI Section Line/RConn2 -- b/RConn1
  Three-Phase PI Section Line/RConn1 -- a/RConn1

== system LV_grid/L22/L1 ==
  Pi Section Line : spsPiSectionLineLib/Pi Section Line  LConnTagsString=__new0  RConnTagsString=__new0  Phases=1  PiSections=1  Length=0.0025  Frequency=50  Resistance=0.274  Inductance=0.073  Capacitance=12.74e-9  Measurements=None  Measurements2=None
      settings: SourceProductBaseCode=PS
  Three-Phase PI Section Line : spsThreePhasePISectionLineLib/Three-Phase PI Section Line  LConnTagsString=a|b|c  RConnTagsString=A|B|C  Length=0.0025  Frequency=50  Resistances=[ 0.274 0.959]  Inductances=[ 0.073 0.079]  Capacitances=[12.74e-9 7.751e-9]
  A : PMIOPort  Side=Left
  B : PMIOPort  Port=2  Side=Left
  C : PMIOPort  Port=3  Side=Left
  N : PMIOPort  Port=4  Side=Left
  a : PMIOPort  Port=5  Side=Right
  b : PMIOPort  Port=6  Side=Right
  c : PMIOPort  Port=7  Side=Right
  n : PMIOPort  Port=8  Side=Right
  connections:
  Pi Section Line/LConn1 -- N/RConn1
  Pi Section Line/RConn1 -- n/RConn1
  C/RConn1 -- Three-Phase PI Section Line/LConn3
  B/RConn1 -- Three-Phase PI Section Line/LConn2
  A/RConn1 -- Three-Phase PI Section Line/LConn1
  Three-Phase PI Section Line/RConn3 -- c/RConn1
  Three-Phase PI Section Line/RConn2 -- b/RConn1
  Three-Phase PI Section Line/RConn1 -- a/RConn1

== system LV_grid/L22/L2 ==
  Pi Section Line : spsPiSectionLineLib/Pi Section Line  LConnTagsString=__new0  RConnTagsString=__new0  Phases=1  PiSections=1  Length=0.0025  Frequency=50  Resistance=0.274  Inductance=0.073  Capacitance=12.74e-9  Measurements=None  Measurements2=None
      settings: SourceProductBaseCode=PS
  Three-Phase PI Section Line : spsThreePhasePISectionLineLib/Three-Phase PI Section Line  LConnTagsString=a|b|c  RConnTagsString=A|B|C  Length=0.0025  Frequency=50  Resistances=[ 0.274 0.959]  Inductances=[ 0.073 0.079]  Capacitances=[12.74e-9 7.751e-9]
  A : PMIOPort  Side=Left
  B : PMIOPort  Port=2  Side=Left
  C : PMIOPort  Port=3  Side=Left
  N : PMIOPort  Port=4  Side=Left
  a : PMIOPort  Port=5  Side=Right
  b : PMIOPort  Port=6  Side=Right
  c : PMIOPort  Port=7  Side=Right
  n : PMIOPort  Port=8  Side=Right
  connections:
  Pi Section Line/LConn1 -- N/RConn1
  Pi Section Line/RConn1 -- n/RConn1
  C/RConn1 -- Three-Phase PI Section Line/LConn3
  B/RConn1 -- Three-Phase PI Section Line/LConn2
  A/RConn1 -- Three-Phase PI Section Line/LConn1
  Three-Phase PI Section Line/RConn3 -- c/RConn1
  Three-Phase PI Section Line/RConn2 -- b/RConn1
  Three-Phase PI Section Line/RConn1 -- a/RConn1

== system LV_grid/L23/L1 ==
  Pi Section Line : spsPiSectionLineLib/Pi Section Line  LConnTagsString=__new0  RConnTagsString=__new0  Phases=1  PiSections=1  Length=0.0025  Frequency=50  Resistance=0.274  Inductance=0.073  Capacitance=12.74e-9  Measurements=None  Measurements2=None
      settings: SourceProductBaseCode=PS
  Three-Phase PI Section Line : spsThreePhasePISectionLineLib/Three-Phase PI Section Line  LConnTagsString=a|b|c  RConnTagsString=A|B|C  Length=0.0025  Frequency=50  Resistances=[ 0.274 0.959]  Inductances=[ 0.073 0.079]  Capacitances=[12.74e-9 7.751e-9]
  A : PMIOPort  Side=Left
  B : PMIOPort  Port=2  Side=Left
  C : PMIOPort  Port=3  Side=Left
  N : PMIOPort  Port=4  Side=Left
  a : PMIOPort  Port=5  Side=Right
  b : PMIOPort  Port=6  Side=Right
  c : PMIOPort  Port=7  Side=Right
  n : PMIOPort  Port=8  Side=Right
  connections:
  Pi Section Line/LConn1 -- N/RConn1
  Pi Section Line/RConn1 -- n/RConn1
  C/RConn1 -- Three-Phase PI Section Line/LConn3
  B/RConn1 -- Three-Phase PI Section Line/LConn2
  A/RConn1 -- Three-Phase PI Section Line/LConn1
  Three-Phase PI Section Line/RConn3 -- c/RConn1
  Three-Phase PI Section Line/RConn2 -- b/RConn1
  Three-Phase PI Section Line/RConn1 -- a/RConn1

== system LV_grid/L23/L2 ==
  Pi Section Line : spsPiSectionLineLib/Pi Section Line  LConnTagsString=__new0  RConnTagsString=__new0  Phases=1  PiSections=1  Length=0.0025  Frequency=50  Resistance=0.274  Inductance=0.073  Capacitance=12.74e-9  Measurements=None  Measurements2=None
      settings: SourceProductBaseCode=PS
  Three-Phase PI Section Line : spsThreePhasePISectionLineLib/Three-Phase PI Section Line  LConnTagsString=a|b|c  RConnTagsString=A|B|C  Length=0.0025  Frequency=50  Resistances=[ 0.274 0.959]  Inductances=[ 0.073 0.079]  Capacitances=[12.74e-9 7.751e-9]
  A : PMIOPort  Side=Left
  B : PMIOPort  Port=2  Side=Left
  C : PMIOPort  Port=3  Side=Left
  N : PMIOPort  Port=4  Side=Left
  a : PMIOPort  Port=5  Side=Right
  b : PMIOPort  Port=6  Side=Right
  c : PMIOPort  Port=7  Side=Right
  n : PMIOPort  Port=8  Side=Right
  connections:
  Pi Section Line/LConn1 -- N/RConn1
  Pi Section Line/RConn1 -- n/RConn1
  C/RConn1 -- Three-Phase PI Section Line/LConn3
  B/RConn1 -- Three-Phase PI Section Line/LConn2
  A/RConn1 -- Three-Phase PI Section Line/LConn1
  Three-Phase PI Section Line/RConn3 -- c/RConn1
  Three-Phase PI Section Line/RConn2 -- b/RConn1
  Three-Phase PI Section Line/RConn1 -- a/RConn1

== system LV_grid/L23/L3 ==
  Pi Section Line : spsPiSectionLineLib/Pi Section Line  LConnTagsString=__new0  RConnTagsString=__new0  Phases=1  PiSections=1  Length=0.0025  Frequency=50  Resistance=0.274  Inductance=0.073  Capacitance=12.74e-9  Measurements=None  Measurements2=None
      settings: SourceProductBaseCode=PS
  Three-Phase PI Section Line : spsThreePhasePISectionLineLib/Three-Phase PI Section Line  LConnTagsString=a|b|c  RConnTagsString=A|B|C  Length=0.0025  Frequency=50  Resistances=[ 0.274 0.959]  Inductances=[ 0.073 0.079]  Capacitances=[12.74e-9 7.751e-9]
  A : PMIOPort  Side=Left
  B : PMIOPort  Port=2  Side=Left
  C : PMIOPort  Port=3  Side=Left
  N : PMIOPort  Port=4  Side=Left
  a : PMIOPort  Port=5  Side=Right
  b : PMIOPort  Port=6  Side=Right
  c : PMIOPort  Port=7  Side=Right
  n : PMIOPort  Port=8  Side=Right
  connections:
  Pi Section Line/LConn1 -- N/RConn1
  Pi Section Line/RConn1 -- n/RConn1
  C/RConn1 -- Three-Phase PI Section Line/LConn3
  B/RConn1 -- Three-Phase PI Section Line/LConn2
  A/RConn1 -- Three-Phase PI Section Line/LConn1
  Three-Phase PI Section Line/RConn3 -- c/RConn1
  Three-Phase PI Section Line/RConn2 -- b/RConn1
  Three-Phase PI Section Line/RConn1 -- a/RConn1

== system LV_grid/L23/L4 ==
  Pi Section Line : spsPiSectionLineLib/Pi Section Line  LConnTagsString=__new0  RConnTagsString=__new0  Phases=1  PiSections=1  Length=0.0025  Frequency=50  Resistance=0.274  Inductance=0.073  Capacitance=12.74e-9  Measurements=None  Measurements2=None
      settings: SourceProductBaseCode=PS
  Three-Phase PI Section Line : spsThreePhasePISectionLineLib/Three-Phase PI Section Line  LConnTagsString=a|b|c  RConnTagsString=A|B|C  Length=0.0025  Frequency=50  Resistances=[ 0.274 0.959]  Inductances=[ 0.073 0.079]  Capacitances=[12.74e-9 7.751e-9]
  A : PMIOPort  Side=Left
  B : PMIOPort  Port=2  Side=Left
  C : PMIOPort  Port=3  Side=Left
  N : PMIOPort  Port=4  Side=Left
  a : PMIOPort  Port=5  Side=Right
  b : PMIOPort  Port=6  Side=Right
  c : PMIOPort  Port=7  Side=Right
  n : PMIOPort  Port=8  Side=Right
  connections:
  Pi Section Line/LConn1 -- N/RConn1
  Pi Section Line/RConn1 -- n/RConn1
  C/RConn1 -- Three-Phase PI Section Line/LConn3
  B/RConn1 -- Three-Phase PI Section Line/LConn2
  A/RConn1 -- Three-Phase PI Section Line/LConn1
  Three-Phase PI Section Line/RConn3 -- c/RConn1
  Three-Phase PI Section Line/RConn2 -- b/RConn1
  Three-Phase PI Section Line/RConn1 -- a/RConn1

== system LV_grid/L23/L5 ==
  Pi Section Line : spsPiSectionLineLib/Pi Section Line  LConnTagsString=__new0  RConnTagsString=__new0  Phases=1  PiSections=1  Length=0.0025  Frequency=50  Resistance=0.274  Inductance=0.073  Capacitance=12.74e-9  Measurements=None  Measurements2=None
      settings: SourceProductBaseCode=PS
  Three-Phase PI Section Line : spsThreePhasePISectionLineLib/Three-Phase PI Section Line  LConnTagsString=a|b|c  RConnTagsString=A|B|C  Length=0.0025  Frequency=50  Resistances=[ 0.274 0.959]  Inductances=[ 0.073 0.079]  Capacitances=[12.74e-9 7.751e-9]
  A : PMIOPort  Side=Left
  B : PMIOPort  Port=2  Side=Left
  C : PMIOPort  Port=3  Side=Left
  N : PMIOPort  Port=4  Side=Left
  a : PMIOPort  Port=5  Side=Right
  b : PMIOPort  Port=6  Side=Right
  c : PMIOPort  Port=7  Side=Right
  n : PMIOPort  Port=8  Side=Right
  connections:
  Pi Section Line/LConn1 -- N/RConn1
  Pi Section Line/RConn1 -- n/RConn1
  C/RConn1 -- Three-Phase PI Section Line/LConn3
  B/RConn1 -- Three-Phase PI Section Line/LConn2
  A/RConn1 -- Three-Phase PI Section Line/LConn1
  Three-Phase PI Section Line/RConn3 -- c/RConn1
  Three-Phase PI Section Line/RConn2 -- b/RConn1
  Three-Phase PI Section Line/RConn1 -- a/RConn1

== system LV_grid/L24/L1 ==
  Pi Section Line : spsPiSectionLineLib/Pi Section Line  LConnTagsString=__new0  RConnTagsString=__new0  Phases=1  PiSections=1  Length=0.0025  Frequency=50  Resistance=0.274  Inductance=0.073  Capacitance=12.74e-9  Measurements=None  Measurements2=None
      settings: SourceProductBaseCode=PS
  Three-Phase PI Section Line : spsThreePhasePISectionLineLib/Three-Phase PI Section Line  LConnTagsString=a|b|c  RConnTagsString=A|B|C  Length=0.0025  Frequency=50  Resistances=[ 0.274 0.959]  Inductances=[ 0.073 0.079]  Capacitances=[12.74e-9 7.751e-9]
  A : PMIOPort  Side=Left
  B : PMIOPort  Port=2  Side=Left
  C : PMIOPort  Port=3  Side=Left
  N : PMIOPort  Port=4  Side=Left
  a : PMIOPort  Port=5  Side=Right
  b : PMIOPort  Port=6  Side=Right
  c : PMIOPort  Port=7  Side=Right
  n : PMIOPort  Port=8  Side=Right
  connections:
  Pi Section Line/LConn1 -- N/RConn1
  Pi Section Line/RConn1 -- n/RConn1
  C/RConn1 -- Three-Phase PI Section Line/LConn3
  B/RConn1 -- Three-Phase PI Section Line/LConn2
  A/RConn1 -- Three-Phase PI Section Line/LConn1
  Three-Phase PI Section Line/RConn3 -- c/RConn1
  Three-Phase PI Section Line/RConn2 -- b/RConn1
  Three-Phase PI Section Line/RConn1 -- a/RConn1

== system LV_grid/L24/L2 ==
  Pi Section Line : spsPiSectionLineLib/Pi Section Line  LConnTagsString=__new0  RConnTagsString=__new0  Phases=1  PiSections=1  Length=0.0025  Frequency=50  Resistance=0.274  Inductance=0.073  Capacitance=12.74e-9  Measurements=None  Measurements2=None
      settings: SourceProductBaseCode=PS
  Three-Phase PI Section Line : spsThreePhasePISectionLineLib/Three-Phase PI Section Line  LConnTagsString=a|b|c  RConnTagsString=A|B|C  Length=0.0025  Frequency=50  Resistances=[ 0.274 0.959]  Inductances=[ 0.073 0.079]  Capacitances=[12.74e-9 7.751e-9]
  A : PMIOPort  Side=Left
  B : PMIOPort  Port=2  Side=Left
  C : PMIOPort  Port=3  Side=Left
  N : PMIOPort  Port=4  Side=Left
  a : PMIOPort  Port=5  Side=Right
  b : PMIOPort  Port=6  Side=Right
  c : PMIOPort  Port=7  Side=Right
  n : PMIOPort  Port=8  Side=Right
  connections:
  Pi Section Line/LConn1 -- N/RConn1
  Pi Section Line/RConn1 -- n/RConn1
  C/RConn1 -- Three-Phase PI Section Line/LConn3
  B/RConn1 -- Three-Phase PI Section Line/LConn2
  A/RConn1 -- Three-Phase PI Section Line/LConn1
  Three-Phase PI Section Line/RConn3 -- c/RConn1
  Three-Phase PI Section Line/RConn2 -- b/RConn1
  Three-Phase PI Section Line/RConn1 -- a/RConn1

== system LV_grid/L24/L3 ==
  Pi Section Line : spsPiSectionLineLib/Pi Section Line  LConnTagsString=__new0  RConnTagsString=__new0  Phases=1  PiSections=1  Length=0.0025  Frequency=50  Resistance=0.274  Inductance=0.073  Capacitance=12.74e-9  Measurements=None  Measurements2=None
      settings: SourceProductBaseCode=PS
  Three-Phase PI Section Line : spsThreePhasePISectionLineLib/Three-Phase PI Section Line  LConnTagsString=a|b|c  RConnTagsString=A|B|C  Length=0.0025  Frequency=50  Resistances=[ 0.274 0.959]  Inductances=[ 0.073 0.079]  Capacitances=[12.74e-9 7.751e-9]
  A : PMIOPort  Side=Left
  B : PMIOPort  Port=2  Side=Left
  C : PMIOPort  Port=3  Side=Left
  N : PMIOPort  Port=4  Side=Left
  a : PMIOPort  Port=5  Side=Right
  b : PMIOPort  Port=6  Side=Right
  c : PMIOPort  Port=7  Side=Right
  n : PMIOPort  Port=8  Side=Right
  connections:
  Pi Section Line/LConn1 -- N/RConn1
  Pi Section Line/RConn1 -- n/RConn1
  C/RConn1 -- Three-Phase PI Section Line/LConn3
  B/RConn1 -- Three-Phase PI Section Line/LConn2
  A/RConn1 -- Three-Phase PI Section Line/LConn1
  Three-Phase PI Section Line/RConn3 -- c/RConn1
  Three-Phase PI Section Line/RConn2 -- b/RConn1
  Three-Phase PI Section Line/RConn1 -- a/RConn1

== system LV_grid/L24/L4 ==
  Pi Section Line : spsPiSectionLineLib/Pi Section Line  LConnTagsString=__new0  RConnTagsString=__new0  Phases=1  PiSections=1  Length=0.0025  Frequency=50  Resistance=0.274  Inductance=0.073  Capacitance=12.74e-9  Measurements=None  Measurements2=None
      settings: SourceProductBaseCode=PS
  Three-Phase PI Section Line : spsThreePhasePISectionLineLib/Three-Phase PI Section Line  LConnTagsString=a|b|c  RConnTagsString=A|B|C  Length=0.0025  Frequency=50  Resistances=[ 0.274 0.959]  Inductances=[ 0.073 0.079]  Capacitances=[12.74e-9 7.751e-9]
  A : PMIOPort  Side=Left
  B : PMIOPort  Port=2  Side=Left
  C : PMIOPort  Port=3  Side=Left
  N : PMIOPort  Port=4  Side=Left
  a : PMIOPort  Port=5  Side=Right
  b : PMIOPort  Port=6  Side=Right
  c : PMIOPort  Port=7  Side=Right
  n : PMIOPort  Port=8  Side=Right
  connections:
  Pi Section Line/LConn1 -- N/RConn1
  Pi Section Line/RConn1 -- n/RConn1
  C/RConn1 -- Three-Phase PI Section Line/LConn3
  B/RConn1 -- Three-Phase PI Section Line/LConn2
  A/RConn1 -- Three-Phase PI Section Line/LConn1
  Three-Phase PI Section Line/RConn3 -- c/RConn1
  Three-Phase PI Section Line/RConn2 -- b/RConn1
  Three-Phase PI Section Line/RConn1 -- a/RConn1
